simulink model "airspeed_hold_using_commanded_pitch"  (Simulink 7.7)
settings: Solver=ode45  StartTime=0.0  StopTime=10.0  RelTol=1e-3
undefined symbols (not defined in the file): a_theta_2, a_theta_3, a_V_1, g, k_i_V_2, k_p_theta, k_p_V_2
settings Model: Creator=prattmic  LastModifiedBy=prattmic

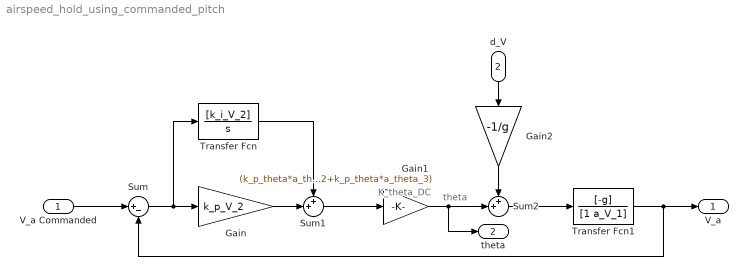
== system airspeed_hold_using_commanded_pitch ==
  note: K_theta_DC
  note: theta
  V_a Commanded : Inport
  d_V : Inport  Port=2
  Gain : Gain  Gain=k_p_V_2
  Gain1 : Gain  Gain=(k_p_theta*a_theta_3)/(a_theta_2+k_p_theta*a_theta_3)
  Gain2 : Gain  Gain=-1/g
  Sum : Sum  Inputs=|+-
  Sum1 : Sum  Inputs=++|
  Sum2 : Sum  Inputs=++|
  Transfer Fcn : TransferFcn  Numerator=[k_i_V_2]  Denominator=[1 0]
  Transfer Fcn1 : TransferFcn  Numerator=[-g]  Denominator=[1 a_V_1]
  V_a : Outport
  theta : Outport  Port=2
  wires:
  d_V/1 -> Gain2/1
  Transfer Fcn/1 -> Sum1/1
  Gain2/1 -> Sum2/1
  V_a Commanded/1 -> Sum/1
  Sum/1 -> Gain/1, Transfer Fcn/1
  Gain/1 -> Sum1/2
  Sum1/1 -> Gain1/1
  Gain1/1 -> Sum2/2, theta/1
  Sum2/1 -> Transfer Fcn1/1
  Transfer Fcn1/1 -> V_a/1, Sum/2
